simulink model "quadcopter_NN"  (R2018b)
settings: Solver=FixedStepAuto  StartTime=0.0  StopTime=options.T_train  FixedStep=options.dt  RelTol=1e-3
undefined symbols (not defined in the file or in its folder): options
libraries: neural x136, simulink x3
(part 6 of 6)

== system quadcopter_NN/ΝΝ_cex_1/Layer 3/Delays 1 ==
  "p{3}" : Inport  PortDimensions=30
      mask Display: e = 0.06;c1 = [120 230 180]/255;c2 = ([120 230 180]+0)/(256+128);c3 = ([120 230 180]+128)/(256+128);patch([0 1 1 0],[0 0 1 1],c1);patch([0 1 1 1-e 1-e 0+e],[0 0 1 1-e 0+e 0+e],c2);patch([0 0 1 1-e 0+e 0+e],[0 1 1 1-e 1-e 0+e],c3);plot([0 1 1 0 0],[0 0 1 1 0]);
  mux : Mux  Inputs=1
      mask Display: e = 0.06;c1 = [120 150 230]/255;c2 = ([120 150 230]+0)/383;c3 = ([120 150 230]+128)/383;patch([0 1 1 0],[0 0 1 1],c1);patch([0 1 1 1-e 1-e 0+e],[0 0 1 1-e 0+e 0+e],c2);patch([0 0 1 1-e 0+e 0+e],[0 1 1 1-e 1-e 0+e],c3);plot([0 1 1 0 0],[0 0 1 1 0]);disp('Mux')
  "pd{3,2}" : Outport
      mask Display: e = 0.06;c1 = [120 230 180]/255;c2 = ([120 230 180]+0)/(256+128);c3 = ([120 230 180]+128)/(256+128);patch([0 1 1 0],[0 0 1 1],c1);patch([0 1 1 1-e 1-e 0+e],[0 0 1 1-e 0+e 0+e],c2);patch([0 0 1 1-e 0+e 0+e],[0 1 1 1-e 1-e 0+e],c3);plot([0 1 1 0 0],[0 0 1 1 0]);
  wires:
  "p{3}"/1 -> mux/1
  mux/1 -> "pd{3,2}"/1

== system quadcopter_NN/ΝΝ_cex_1/Layer 3/LW{3,2} ==
  "ad{3,2}" : Inport  PortDimensions=30
      mask Display: e = 0.06;c1 = [120 230 180]/255;c2 = ([120 230 180]+0)/(256+128);c3 = ([120 230 180]+128)/(256+128);patch([0 1 1 0],[0 0 1 1],c1);patch([0 1 1 1-e 1-e 0+e],[0 0 1 1-e 0+e 0+e],c2);patch([0 0 1 1-e 0+e 0+e],[0 1 1 1-e 1-e 0+e],c3);plot([0 1 1 0 0],[0 0 1 1 0]);
  "IW{3,2}(1,:)'" : Constant  Value=[0.28605281370942170493520961827016435563564300537109375;0.280558170768164416575274344722856767475605010986328125;-0.04465182592316856158287663447481463663280010223388671875;-0.185057175926483130634636609102017246186733245849609375;-0.201806834550275426831689173923223279416561126708984375;-0.053901188667638440243923270145387505181133747100830078125;0.28350795514972981781198768658214248716831207275390625;-0.1373883202951985127437950495732366107404232025146484375;-0.1434300080792637877014072955716983415186405181884765625;0.164760392329380500608948523222352378070354461669921875;0.170816328822324836611556975185521878302097320556640625;0.0905435547260626527599214341535116545855998992919921875;0.32592151189934603916498190301354043185710906982421875;0.157816289822740929427169476184644736349582672119140625;0.280142536820981946643627225057571195065975189208984375;-0.097490414502118649675566075529786758124828338623046875;-0.19463861024315132208784007161739282310009002685546875;-0.1898121343732174504115306490348302759230136871337890625;-0.1740230658061422130966633403659216128289699554443359375;0.05667112035554992821584363582587684504687786102294921875;-0.08765572647923834670447007511029369197785854339599609375;-0.3234856378299217904981333049363456666469573974609375;0.31135815253106791100634609392727725207805633544921875;0.301052719859545125924427111385739408433437347412109375;-0.2062094874504673824855416341961245052516460418701171875;-0.314040758678562514916166037437506020069122314453125;-0.1929878711611880126586271444466547109186649322509765625;-0.2731142892781084352549214600003324449062347412109375;0.31074483876510072821730545911123044788837432861328125;0.383478552002913419816110263127484358847141265869140625]
      mask Display: e = 0.06;c1 = [120 150 230]/255;c2 = ([120 150 230]+0)/383;c3 = ([120 150 230]+128)/383;patch([0 1 1 0],[0 0 1 1],c1);patch([0 1 1 1-e 1-e 0+e],[0 0 1 1-e 0+e 0+e],c2);patch([0 0 1 1-e 0+e 0+e],[0 1 1 1-e 1-e 0+e],c3);plot([0 1 1 0 0],[0 0 1 1 0]);disp('weights');
  Mux : Mux  Inputs=1
      mask Display: e = 0.06;c1 = [120 150 230]/255;c2 = ([120 150 230]+0)/383;c3 = ([120 150 230]+128)/383;patch([0 1 1 0],[0 0 1 1],c1);patch([0 1 1 1-e 1-e 0+e],[0 0 1 1-e 0+e 0+e],c2);patch([0 0 1 1-e 0+e 0+e],[0 1 1 1-e 1-e 0+e],c3);plot([0 1 1 0 0],[0 0 1 1 0]);disp('Mux');
  dotprod1 : neural/Weight Functions/dotprod
  "lz{3,2}" : Outport
      mask Display: e = 0.06;c1 = [120 230 180]/255;c2 = ([120 230 180]+0)/(256+128);c3 = ([120 230 180]+128)/(256+128);patch([0 1 1 0],[0 0 1 1],c1);patch([0 1 1 1-e 1-e 0+e],[0 0 1 1-e 0+e 0+e],c2);patch([0 0 1 1-e 0+e 0+e],[0 1 1 1-e 1-e 0+e],c3);plot([0 1 1 0 0],[0 0 1 1 0]);
  wires:
  "IW{3,2}(1,:)'"/1 -> dotprod1/1
  "ad{3,2}"/1 -> dotprod1/2
  dotprod1/1 -> Mux/1
  Mux/1 -> "lz{3,2}"/1

== matlab function quadcopter_NN/MATLAB Function ==
  data: r1 input; F output; r2 input; r3 input; x3 input; x6 input; x7 input; x8 input; x10 input; x11 input; tau_phi output; tau_theta output; tau_psi output
function [F,tau_phi,tau_theta,tau_psi] = fcn(r1,r2,r3,x3,x6,x7,x8,x10,x11)
%initialization
m=1.4;
g=9.81;
F= m*g-10*(x3-r1)+3*x6;
tau_phi=-(x7-r2)-x10;
tau_theta=-(x8-r3)-x11;
tau_psi=0;
